simulink model "servo_motor"  (R2014a)
settings: Solver=ode15s  StartTime=0.0  StopTime=0.2  RelTol=1e-3
values from neighbouring files (symbols this model uses):
  b = 3.5077e-6    (= 3.5077e-06)    [servo.m]
  J = 3.2284e-6    (= 3.2284e-06)    [servo.m]
  K = 0.0274    [servo.m]
  L = 2.75e-6    (= 2.75e-06)    [servo.m]
  R = 4    [servo.m]
settings Model: Creator=JinilGondalia  LastModifiedBy=JinilGondalia

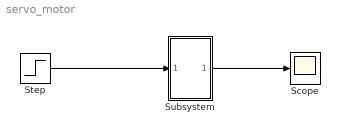
== system servo_motor ==
  Scope : Scope
  Step : Step  Time=0.1  SampleTime=0
  Subsystem : Subsystem
  wires:
  Step/1 -> Subsystem/1(In1)
  Subsystem/1(Out1) -> Scope/1

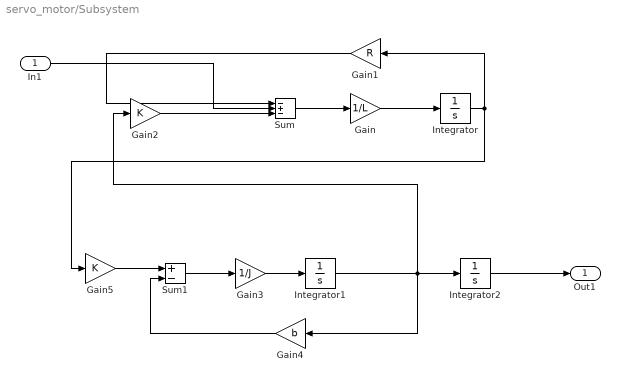
== system servo_motor/Subsystem ==
  In1 : Inport
  Gain : Gain  Gain=1/L
  Gain1 : Gain  Gain=R
  Gain2 : Gain  Gain=K
  Gain3 : Gain  Gain=1/J
  Gain4 : Gain  Gain=b
  Gain5 : Gain  Gain=K
  Integrator : Integrator
  Integrator1 : Integrator
  Integrator2 : Integrator
  Sum : Sum  Inputs=-+-
  Sum1 : Sum  Inputs=+-
  Out1 : Outport
  wires:
  Gain4/1 -> Sum1/2
  In1/1 -> Sum/2
  Gain2/1 -> Sum/3
  Integrator/1 -> Gain5/1, Gain1/1
  Gain1/1 -> Sum/1
  Gain/1 -> Integrator/1
  Sum/1 -> Gain/1
  Integrator1/1 -> Gain4/1, Gain2/1, Integrator2/1
  Gain3/1 -> Integrator1/1
  Sum1/1 -> Gain3/1
  Gain5/1 -> Sum1/1
  Integrator2/1 -> Out1/1
